simulink model "ADRC"  (R2022b)
settings: Solver=FixedStepAuto  StartTime=0.0  StopTime=10.0  FixedStep=0.01  RelTol=1e-3
values from neighbouring files (symbols this model uses):
  b = 1    [ini.m]
settings Model: Creator=张倬境  LastModifiedBy=张倬境

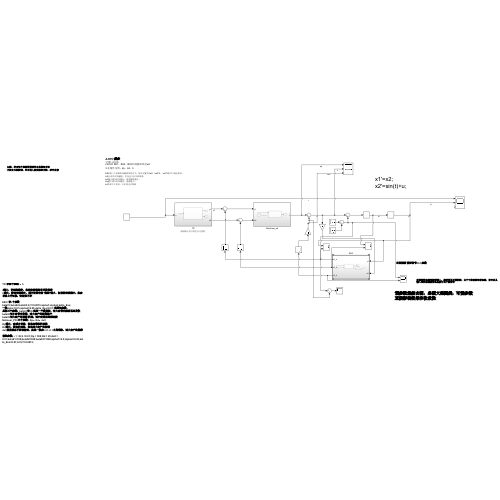
[thumbnail: Simulink's stored preview of the top-level diagram]
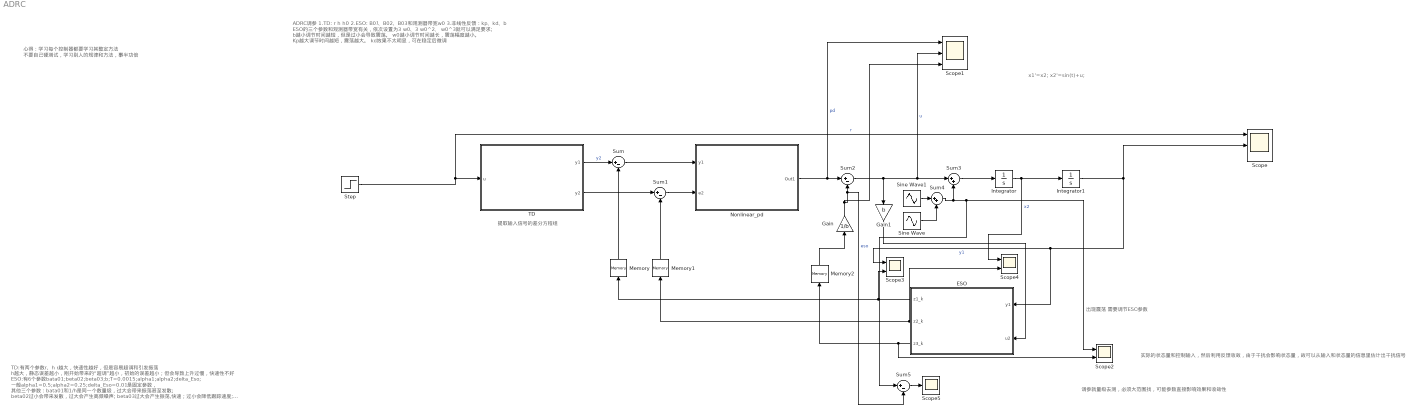
== system ADRC ==
  note: TD:有两个参数r、h
      |
      | r越大，快速性越好，但是容易超调和引发振荡
      | h越大，静态误差越小，刚开始带来的“超调”越小，初始的误差越小；但会导致上升过慢，快速性不好
      |
      | ESO:有6个参数bata01;beta02;beta03;b;T=0.0015;alpha1;alpha2;delta_Eso;
      | 一般alpha1=0.5;alpha2=0.25;delta_Eso=0.01;是固定参数，
      | 其他三个参数：bata01和1/h是同一个数量级，过大会带来振荡甚至发散;
      | beta02过小会带来发散，过大会产生高频噪声;
      | beta03过大会产生振荡,快速；过小会降低跟踪速度;
      | Nolinear_PD:三个参数：Kp、Kd、delt
      | Kp越大，会减少误差，但是会降低快速性
      | Kd越大，增加快速性，但是过大会产生振荡
      | delt的值基本不影响输出，但是一般在0.01~0.1之间选取，过大会产生振荡
      |
      | 最终参数：r = 30;h =0.01;Kp = 500;Kd = 25;delt = 0.01;bata01=100;beta02=300;beta03=1500;alpha1=0.5;alpha2=0.25;delta_Eso=0.01;b=5;T=0.0015;
  note: 心得：学习每个控制器都要学习其整定方法
      | 不要自己硬测试，学习别人的规律和方法，事半功倍
  note: ADRC调参
      | 1.TD: r h h0
      | 2.ESO: B01、B02、B03和观测器带宽w0
      | 3.非线性反馈：kp、kd、b
      |
      | ESO的三个参数和观测器带宽有关，依次设置为3 w0、3 w0^2、 w0^3就可以满足要求;
      | b越小调节时间越短，但是过小会导致震荡。
      | w0越小调节时间越长，震荡幅度越小。
      | Kp越大调节时间越短，震荡越大。
      | kd效果不太明显，可在稳定后微调
  note: 调参就量级去测，必须大范围找，可能参数直接影响效果和收敛性
  note: 实际的状态量和控制输入，然后利用反馈收敛，由于干扰会影响状态量，故可以从输入和状态量的信息里估计出干扰信号
  note: x1'=x2;
      | x2'=sin(t)+u;
  note: 出现震荡 需要调节ESO参数
  note: 提取输入信号的差分方程组
  ESO : Subsystem
  Gain : Gain  Gain=1/b
  Gain1 : Gain  Gain=b
  Integrator : Integrator
  Integrator1 : Integrator
  Memory : Memory
  Memory1 : Memory
  Memory2 : Memory
  Nonlinear_pd : Subsystem
  Scope : Scope  NumInputPorts=3
  Scope1 : Scope  NumInputPorts=3
  Scope2 : Scope  NumInputPorts=2
  Scope3 : Scope  NumInputPorts=2
  Scope4 : Scope  NumInputPorts=2
  Scope5 : Scope
  Sine Wave : Sin  SampleTime=0
  Sine Wave1 : Sin  Frequency=2  Phase=pi/2  SampleTime=0
  Step : Step  SampleTime=0
  Sum{,1..2,5} (4 alike) : Sum  Inputs=|+-
  Sum3 : Sum  Inputs=|++
  Sum4 : Sum  Inputs=|++
  TD : Subsystem
  wires:
  TD/1(y1) -> Sum/1  "y2"
  Sum/1 -> Nonlinear_pd/1(y1)
  TD/2(y2) -> Sum1/1
  Sum1/1 -> Nonlinear_pd/2(e2)
  ESO/3(z3_k) -> Scope2/2, Memory2/1
  Sum2/1 -> Scope1/2, Sum3/1, Gain1/1  "u"
  Sum3/1 -> Integrator/1
  Integrator1/1 -> Scope/2, Scope3/1, ESO/1(y1)  "y1"
  Gain1/1 -> ESO/2(u2)
  Step/1 -> Scope/1, TD/1(u)  "r"
  Memory/1 -> Sum/2
  Memory1/1 -> Sum1/2
  Memory2/1 -> Gain/1
  ESO/1(z1_k) -> Scope3/2, Memory/1
  ESO/2(z2_k) -> Memory1/1, Scope4/2
  Integrator/1 -> Scope4/1, Integrator1/1  "x2"
  Sine Wave/1 -> Sum4/2
  Sum4/1 -> Sum3/2, Sum5/1, Scope2/1
  Sine Wave1/1 -> Sum4/1
  Gain/1 -> Sum2/2, Sum5/2, Scope1/3  "eso"
  Nonlinear_pd/1(Out1) -> Scope1/1, Sum2/1  "pd"
  Sum5/1 -> Scope5/1

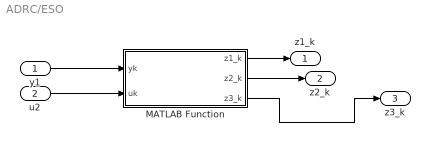
== system ADRC/ESO ==
  y1 : Inport
  u2 : Inport  Port=2
  MATLAB Function : MATLAB Function  TreatAsAtomicUnit=on
  z1_k : Outport
  z2_k : Outport  Port=2
  z3_k : Outport  Port=3
  wires:
  y1/1 -> MATLAB Function/1(yk)
  MATLAB Function/1(z1_k) -> z1_k/1
  u2/1 -> MATLAB Function/2(uk)
  MATLAB Function/2(z2_k) -> z2_k/1
  MATLAB Function/3(z3_k) -> z3_k/1

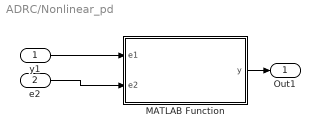
== system ADRC/Nonlinear_pd ==
  y1 : Inport
  e2 : Inport  Port=2
  MATLAB Function : MATLAB Function  TreatAsAtomicUnit=on
  Out1 : Outport
  wires:
  y1/1 -> MATLAB Function/1(e1)
  MATLAB Function/1(y) -> Out1/1
  e2/1 -> MATLAB Function/2(e2)

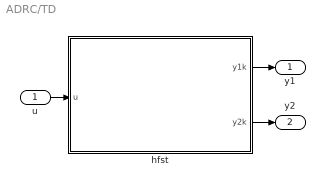
== system ADRC/TD ==
  u : Inport
  hfst : MATLAB Function  TreatAsAtomicUnit=on  SystemSampleTime=0.01
  y1 : Outport
  y2 : Outport  Port=2
  wires:
  u/1 -> hfst/1(u)
  hfst/1(y1k) -> y1/1
  hfst/2(y2k) -> y2/1

== matlab function ADRC/Nonlinear_pd/MATLAB Function ==
  data: e1 input; y output; e2 input
function y =nonlinear_pd(e1,e2)
alfa1=0.75;
alfa2=1.5;
delta=0.2;
beta1=15;
beta2=5;
fal1=1;
fal2=1;


if abs(e1)<=delta
    fal1=e1/(delta^(1-alfa1));
end


if abs(e1)>delta
    fal1=(abs(e1))^(alfa1)*sign(e1);
end


if abs(e2)<=delta
    fal2=e2/(delta^(1-alfa2));
end


if abs(e2)>delta
    fal2=(abs(e2))^(alfa2)*sign(e2);
end


y=beta1*fal1+beta2*fal2;
end

== matlab function ADRC/TD/hfst ==
  data: u input; y1k output; y2k output
function [y1k,y2k] = fcn(u)
persistent y1k_1 y2k_1
h=0.01;
delta=10;
if isempty(y1k_1)
    y1k_1=0;
end


if isempty(y2k_1)
    y2k_1=0;
end


y1k=y1k_1+h*y2k_1;


% hfst计算内容
d=delta*h;
d0=h*d;
y=y1k_1-u+h*y2k_1;
a0=sqrt(d*d+8*delta*abs(y));
a=0;
out1=0;
if abs(y)>d0
    a=y2k_1+(a0-d)/2*sign(y);
end


if abs(y)<=d0
    a=y2k_1+y/h;
end


if abs(a)>d
    out1=-delta*sign(a);
end


if abs(a)<=d
    out1=-delta*a/d;
end
out=out1;
% 更新变量
y2k=y2k_1+h*out;


y1k_1=y1k;
y2k_1=y2k;


end

== matlab function ADRC/ESO/MATLAB Function ==
  settings: updateMethod=DISCRETE
  data: yk input; z1_k output; uk input; z2_k output; z3_k output
function [z1_k,z2_k,z3_k] = ESO(yk,uk)
%%参数初始化
persistent  z1_k_1 z2_k_1 z3_k_1
bata01=100;%大了反而慢
beta02=150;%大了 幅值变小
beta03=3000;%大了 幅值变大一定 快


% W0=33;
% bata01=3*W0;%
% beta02=3*W0*W0;%大 幅值小
% beta03=W0*W0*W0;%大 速度快
h=0.01;
alfa1=0.25;
alfa2=0.5;
delta=0.05;%太小会导致控制量发散
fal1=1;
fal2=1;
if isempty(z1_k_1)
    z1_k_1=0;
end
if isempty(z2_k_1)
    z2_k_1=0;
end
if isempty(z3_k_1)
    z3_k_1=0;
end


e1=z1_k_1-yk;
% e2=z2_k_1-uk;
z1_k=z1_k_1+h*(z2_k_1-bata01*e1);%
z1_k_1=z1_k; %%迭代更新z1_k_1


%%计算fal函数
if abs(e1)<=delta
    fal1=e1/(delta^(1-alfa1));
end
if abs(e1)>delta
    fal1=(abs(e1))^(alfa1)*sign(e1);
end

if abs(e1)<=delta
    fal2=e1/(delta^(1-alfa2));
end
if abs(e1)>delta
    fal2=(abs(e1))^(alfa2)*sign(e1);
end


% z2_k=z2_k_1+h*(z3_k_1+b*uk-beta02*fal1);%此处uk前面有b，simulink uk输入通道1
z2_k=z2_k_1+h*(z3_k_1+uk-beta02*fal1);%此处uk前无b，simulink uk输入通道B
z2_k_1=z2_k;%%迭代更新z2_k_1


z3_k=z3_k_1-h*beta03*fal2;
z3_k_1=z3_k;%%迭代更新z3_k_1


end
